simulink model "Prob4"  (R2020b)
settings: Solver=VariableStepAuto  StartTime=0.0  StopTime=10.0  RelTol=1e-3
settings Model: Creator=shoun  LastModifiedBy=shoun

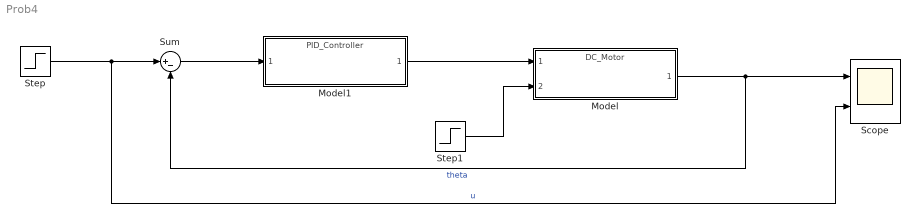
== system Prob4 ==
  Model : ModelReference  ModelNameDialog=DC_Motor.slx  SimulationMode=Normal  ModelReferenceVersion=1.1
  Model1 : ModelReference  ModelNameDialog=PID_Controller.slx  SimulationMode=Normal  ModelReferenceVersion=1.1
  Scope : Scope  NumInputPorts=2
  Step : Step  SampleTime=0
  Step1 : Step  SampleTime=0
  Sum : Sum  Inputs=|+-
  wires:
  Model1/1 -> Model/1
  Step1/1 -> Model/2
  Step/1 -> Scope/2, Sum/1  "u"
  Sum/1 -> Model1/1
  Model/1 -> Sum/2, Scope/1  "theta"
